simulink library "exampleController_cl"  (R2018b)
settings: Solver=VariableStepAuto  StartTime=0.0  StopTime=10.0  RelTol=1e-3
settings Model: Creator=mcobb  LastModifiedBy=mcobb

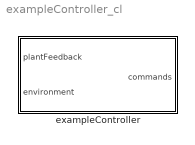
== system exampleController_cl ==
  exampleController : Subsystem

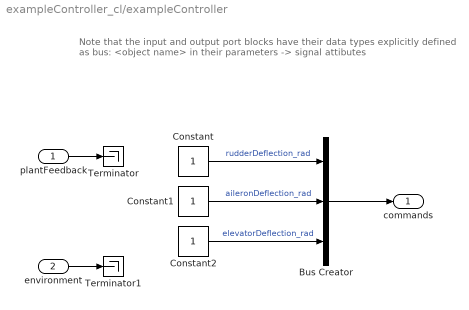
== system exampleController_cl/exampleController ==
  note: Note that the input and output port blocks have their data types
      | explicitly defined as bus: <object name> in their parameters -> signal attibutes
  plantFeedback : Inport  OutDataTypeStr=Bus: plantBus
  environment : Inport  Port=2  OutDataTypeStr=Bus: envBus
  Bus Creator : BusCreator  Inputs=3
  Constant : Constant
  Constant1 : Constant
  Constant2 : Constant
  Terminator : Terminator
  Terminator1 : Terminator
  commands : Outport  OutDataTypeStr=Bus: ctrlBus
  wires:
  plantFeedback/1 -> Terminator/1
  environment/1 -> Terminator1/1
  Bus Creator/1 -> commands/1
  Constant/1 -> Bus Creator/1  "rudderDeflection_rad"
  Constant2/1 -> Bus Creator/3  "elevatorDeflection_rad"
  Constant1/1 -> Bus Creator/2  "aileronDeflection_rad"
